simulink model "csu_ptc_gimbal_actuator_command"  (R2015b)
settings: Solver=VariableStepAuto  StartTime=0.0  StopTime=10.0  RelTol=1e-3
settings Model: Creator=jimkaidy  LastModifiedBy=jimkaidy

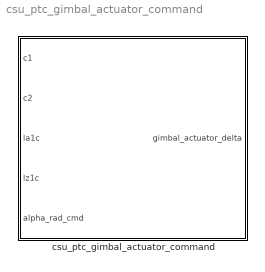
== system csu_ptc_gimbal_actuator_command ==
  csu_ptc_gimbal_actuator_command : MATLAB Function  TreatAsAtomicUnit=on

== matlab function csu_ptc_gimbal_actuator_command/csu_ptc_gimbal_actuator_command ==
  data: c1 input; gimbal_actuator_delta output; c2 input; la1c input; lz1c input; alpha_rad_cmd input
function gimbal_actuator_delta = gimbal_command(c1,c2,la1c,lz1c,alpha_rad_cmd)
%#codegen

Rmount = sqrt(c1^2 + c2^2);

Lcmd = sqrt((la1c - Rmount*sqrt(1 - 1/(1+(tan(alpha_rad_cmd) + c1/c2)^2)))^2 + (lz1c + Rmount/sqrt(1+(tan(alpha_rad_cmd)+c1/c2)^2))^2);

Lo = sqrt((la1c - c1)^2 + (lz1c + c2)^2);

Lerr =( Lcmd - Lo);

gimbal_actuator_delta = Lerr;
